simulink model "HM_to_Unity_2013a"  (R2013a)
settings: Solver=FixedStepDiscrete  StartTime=0.0  StopTime=Inf  FixedStep=0.0004  RelTol=1e-3
InitFcn:
  | SampleTime = 0.0004;
  | sampleTime = 0.0004;
undefined symbols (not defined in the file or in its folder): DiscIntNeverNeededParam
libraries: simulink x26, dspsigops x10, xpcmeasurementcomputinglib x7, xpclib x6, dspmtrx3 x4, etargetslib x2, hm_iointerface_lib x2, hm_control_lib x2, sensors_jr3_lib x1
(part 1 of 2)
settings Model: SimulationMode=external  BufferReuse=off  Creator=janezp  LastModifiedBy=student
settings DataIOCC: LimitDataPoints=off  MaxDataPoints=5000000  SaveFormat=Structure  SignalLoggingSaveFormat=ModelDataLogs  SignalLogging=off  SaveTime=off
settings OptimizationCC: BlockReduction=off  OptimizeBlockIOStorage=off  BufferReuse=off  ExpressionFolding=off  ExpressionDepthLimit=2147483647  LocalBlockOutputs=off  InitFltsAndDblsToZero=on
settings DebuggingCC: SaveWithParameterizedLinksMsg=none  SignalResolutionControl=TryResolveAllWithWarning  MultiTaskDSMMsg=warning  MultiTaskCondExecSysMsg=none  FcnCallInpInsideContextMsg=UseLocalSettings  StrictBusMsg=None
settings HardwareCC: ProdIntDivRoundTo=Zero  ProdEndianess=LittleEndian  ProdHWDeviceType=Generic->32-bit x86 compatible
settings RTWCC: SystemTargetFile=xpctarget.tlc  TemplateMakefile=xpc_default_tmf  Description=xPC Target  ProcessScript=xpctarget_make_rtw_hook  IncludeERTFirstTime=on  RTWCompilerOptimization=On
settings xpcTargetCC: TargetFcnLib=ansi_tfl_table_tmw.mat  CodeReplacementLibrary=XPC_BLAS  ParMdlRefBuildCompliant=on  ConcurrentExecutionCompliant=on  CombineSignalStateStructs=off  MATLABClassNameForMDSCustomization=xpcAperiodicCustomization  GRTInterface=on  GenerateAllocFcn=off  RL32LogTETModifier=off  RL32LogBufSizeModifier=5000000  xPCTaskExecutionProfile=off  xPCRL32EventNumber=5000  xPCLoadParamSetFile=off  xPCConcurrentTasks=off  xPCEnableSFAnimation=off

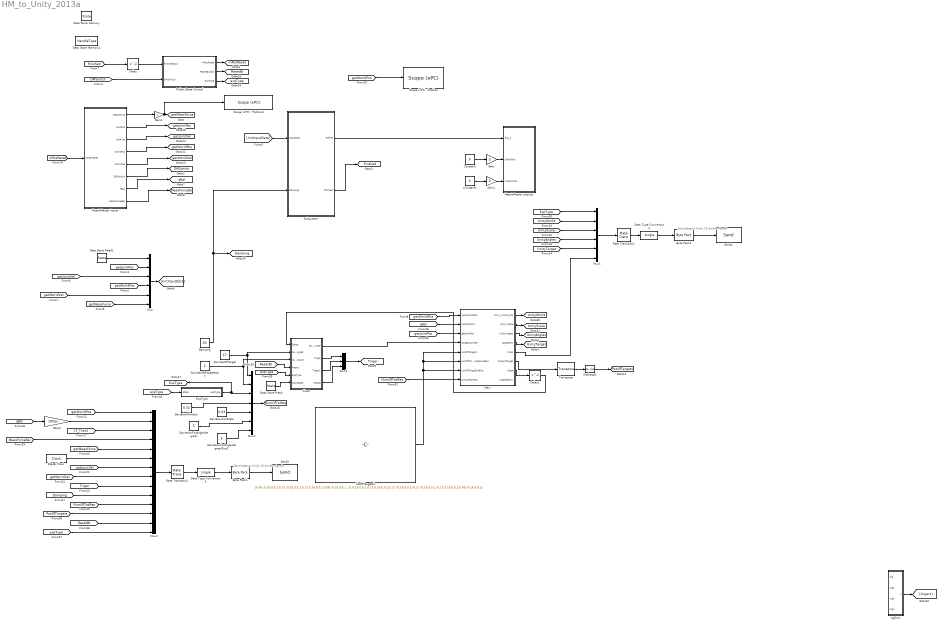
== system HM_to_Unity_2013a ==
  note: Send data to Unity
      | 16 double signals
  note: Send data to Unity
      | 16 double signals
  Byte Pack1 : etargetslib/Byte Pack  datatypes={'single'}  byteAlign=1
  Byte Pack2 : etargetslib/Byte Pack  datatypes={'single'}  byteAlign=1
  Chart : Stateflow chart  TreatAsAtomicUnit=on
  Constant : Constant  Value=0  SampleTime=-1
  Constant1 : Constant  Value=0  SampleTime=-1
  Damping : Constant  Value=40
  Data Store Memory : DataStoreMemory  DataStoreName=State  ReadBeforeWriteMsg=warning  WriteAfterWriteMsg=warning  WriteAfterReadMsg=warning
  Data Store Memory1 : DataStoreMemory  DataStoreName=HandleType  ReadBeforeWriteMsg=warning  WriteAfterWriteMsg=warning  WriteAfterReadMsg=warning
  Data Store Read : DataStoreRead  DataStoreName=State
  Data Store Read1 : DataStoreRead  DataStoreName=State  SampleTime=SampleTime
  Data Type Conversion2 : DataTypeConversion  OutDataTypeStr=single
  Data Type Conversion3 : DataTypeConversion  OutDataTypeStr=single
  Delay : Delay  DelayLength=1  InitialCondition=0
  Delay1 : Delay  DelayLength=1  InitialCondition=0  SampleTime=0.0004
  DeviationForAngle(degree) : Constant  Value=5
  DeviationForAngle(degree)Exp2 : Constant  Value=5
  DeviationForScale : Constant  Value=0.03
  DeviationWindow : Constant  Value=0.02
  Digital Clock : DigitalClock  SampleTime=0.0004
  ExpType : Stateflow chart  TreatAsAtomicUnit=on
  Gain : Gain  Gain=0
  Gain1 : Gain  Gain=0
  Gain2 : Gain
  Gain3 : Gain  Gain=180/pi
  HapticMaster inputs : Subsystem
  HapticMaster outputs : Subsystem
  ListOfTargets1 : Constant  Value=[0.00,-0.16,0,0,1;0.17,-0.16,0,0,1;0.17,0.16,0,0,1;0.00,-0.16,0,0,1;-0.17,-0.16,0,0,1;0.17,-0.16,0,0,1;0.00,-0.16,0,0,1;-0.17,0.16,0,0,1;-0.17,-0.16,0,0,1;0.00,-0.16,0,0,1;0.00,0.16,0,0,1;0.00,-0.16,0,0,1;0.17,0.16,0,0,1;0.17,-0.16,0,0,1;-0.17,-0.16,0,0,1;-0.17,0.16,0,0,1;0.00,-0.16,0,0,1]
  Main : MATLAB Function  TreatAsAtomicUnit=on
  Mux : Mux  Inputs=6
  Mux1 : Mux  Inputs=6
  Mux2 : Mux  Inputs=14
  Mux3 : Mux  Inputs=3
  Mux4 : Mux  Inputs=7
  NumberOfRepeatation : Constant  Value=2
  NumberOfTarget : Constant  Value=17
  Rate Transition1 : RateTransition  OutPortSampleTime=0.02
  Rate Transition2 : RateTransition  OutPortSampleTime=0.01
  Reshape1 : Reshape
  Robot State Control : Subsystem
  Scope (xPC)  Position : xpclib/Misc./Scope (xPC)   scopeno=1  scopetype=Target  autostart=on  viewmode=Numerical  formatstr='Position x: %8.3f m,Position y: %8.3f m,Position z: %8.3f m'  grid=on  ylimits=[0,0]  nosamples=250  noprepostsamples=0  interleave=1  triggermode=FreeRun  triggersignal=1  trigsignalfromport=off  triggerlevel=0.0  triggerslope=Either  triggerscope=1  triggersample=0  filename=data.dat  mode=Lazy  writesize=512  autorestart=off  dynamicfilemode=off  maxwritefilesize=512*1024^2
  Scope (xPC)  Position1 : xpclib/Misc./Scope (xPC)   scopeno=4  scopetype=Target  autostart=on  viewmode=Numerical  formatstr='Fx: %8.3f N,Fy: %8.3f N,Fz: %8.3f N'  grid=on  ylimits=[0,0]  nosamples=250  noprepostsamples=0  interleave=1  triggermode=FreeRun  triggersignal=1  trigsignalfromport=off  triggerlevel=0.0  triggerslope=Either  triggerscope=1  triggersample=0  filename=data.dat  mode=Lazy  writesize=512  autorestart=off  dynamicfilemode=off  maxwritefilesize=512*1024^2
  Send1 : xpclib/UDP/Send  ipAddress=192.168.65.40  ipPort=25008  localPort=-1  vblLen=off  sampletime=0.02
  Send2 : xpclib/UDP/Send  ipAddress=192.168.65.40  ipPort=25010  localPort=-1  vblLen=off  sampletime=0.01
  Subsystem : Subsystem
  Transpose : dspmtrx3/Transpose  Hermitian=off  overflowFlag=off
  "trgSum " : MATLAB Function  TreatAsAtomicUnit=on
  tag scope: DMSwitch=global, Damping=global, ExpType=global, MeasForceBal=global, NumOfTatRep=global, PosOfTargets=global, ResetBt=global, Triger=global, UnityAngles=global, UnityScale=global, UnityTarget=global, UnityWorld=global, expType=global, finished=global, getJointPos=global, getJointVel=global, getMeasForce=global, getWorldPos=global, getWorldVel=global, inPosReset=global, qBal=global
  wires:
  [getWorldPos] -> Mux/4
  [getJointPos] -> Mux/2
  Data Store Read1/1 -> Mux/1
  Mux/1 -> [InitInputData]
  [getWorldPos] -> Scope (xPC)  Position/1
  HapticMaster inputs/1(MeasForce) -> Gain2/1
  HapticMaster inputs/3(JointVel) -> [getJointVel]
  HapticMaster inputs/5(WorldVel) -> [getWorldVel]
  Delay/1 -> Robot State Control/1(finishedTask)
  [DMSwitch] -> Robot State Control/2(DMSwitch)
  Robot State Control/1(inPosReset) -> [inPosReset]
  HapticMaster inputs/6(DMSwitch) -> [DMSwitch]
  [inPosReset] -> HapticMaster inputs/1(inPosReset)
  [getMeasForce] -> Mux/6
  [InitInputData] -> Subsystem/1(InputData)
  Subsystem/2(finished) -> [finished]
  [finished] -> Delay/1
  Subsystem/1(RefVel) -> HapticMaster outputs/1(dot_q)
  HapticMaster inputs/8(MeasForceBal) -> [MeasForceBal]
  HapticMaster inputs/7(qBal) -> [qBal]
  Gain2/1 -> Scope (xPC)  Position1/1, [getMeasForce]
  HapticMaster inputs/4(WorldPos) -> [getWorldPos]
  HapticMaster inputs/2(JointPos) -> [getJointPos]
  [getJointVel] -> Mux/3
  [getWorldVel] -> Mux/5
  "trgSum "/1(y) -> [trigers]
  Rate Transition1/1 -> Data Type Conversion2/1
  Data Type Conversion2/1 -> Byte Pack2/1
  Mux1/1 -> Rate Transition1/1
  Byte Pack2/1 -> Send1/1
  [getWorldPos] -> Main/1(inputWorldPos)
  Main/1(Unity_World_Pos) -> [UnityWorld]
  [UnityWorld] -> Mux1/2
  Main/2(Unity_Scale) -> [UnityScale]
  [UnityScale] -> Mux1/3
  Main/3(UnityAngles) -> [UnityAngles]
  [UnityAngles] -> Mux1/4
  Chart/1(TargetNumber) -> Main/4(TargetNumber)
  Main/4(TargetPos) -> [UnityTarget]
  [UnityTarget] -> Mux1/5
  Main/7(State) -> Delay1/1
  Delay1/1 -> Chart/1(State)
  Main/5(Color) -> Mux1/6
  NumberOfRepeatation/1 -> Mux4/2, Chart/3(NumberOfRepetation)
  NumberOfTarget/1 -> Chart/2(NumOfTarget), Mux4/1
  [getWorldPos] -> Mux2/1
  [qBal] -> Gain3/1
  Gain3/1 -> Mux2/2
  [F_Traw] -> Mux2/3
  [MeasForceBal] -> Mux2/4
  [getMeasForce] -> Mux2/5
  Digital Clock/1 -> Mux2/6
  [getJointVel] -> Mux2/7
  [getWorldVel] -> Mux2/8
  Rate Transition2/1 -> Data Type Conversion3/1
  Byte Pack1/1 -> Send2/1
  Data Type Conversion3/1 -> Byte Pack1/1
  Mux2/1 -> Rate Transition2/1
  [qBal] -> Main/2(inputMotors)
  Chart/2(Triger) -> Mux3/1
  Chart/3(Triger2) -> Mux3/2
  Mux3/1 -> [Triger]
  [Triger] -> Mux2/9
  Mux4/1 -> [NumOfTatRep]
  [NumOfTatRep] -> Main/8(NumOfTarRep)
  [Damping] -> Mux2/10
  Damping/1 -> [Damping], Subsystem/2("Damping ")
  Chart/4(repeat) -> Mux3/3
  [NumOfTatRep] -> Mux2/11
  [PosOfTargets] -> Mux2/12
  Reshape1/1 -> [PosOfTargets]
  Transpose/1 -> Reshape1/1
  Main/6(OutputTarget) -> Transpose/1
  DeviationWindow/1 -> Mux4/4
  [ExpType] -> Mux1/1
  DeviationForScale/1 -> Mux4/5
  DeviationForAngle(degree)/1 -> Mux4/6
  DeviationForAngle(degree)Exp2/1 -> Mux4/7
  [getJointPos] -> Main/3(getJointPos)
  Robot State Control/2("ResetButton ") -> [ResetBt]
  [ResetBt] -> Chart/4(Reset)
  Robot State Control/3(expType) -> [expType]
  [expType] -> ExpType/1(State)
  [expType] -> Chart/5(ExpType)
  [ResetBt] -> Mux2/13
  [expType] -> Mux2/14
  ExpType/1(expType) -> Mux4/3, [ExpType]
  Data Store Read/1 -> Chart/6(MainState)
  ListOfTargets1/1 -> Main/7(ListOfTarget3rdExp), Main/5(ListOfTargets), Main/6(ListOfTargetsForSecondExp)
  Gain/1 -> HapticMaster outputs/2(UMaliMot)
  Constant/1 -> Gain/1
  Constant1/1 -> Gain1/1
  Gain1/1 -> HapticMaster outputs/3(UVelikiMot)

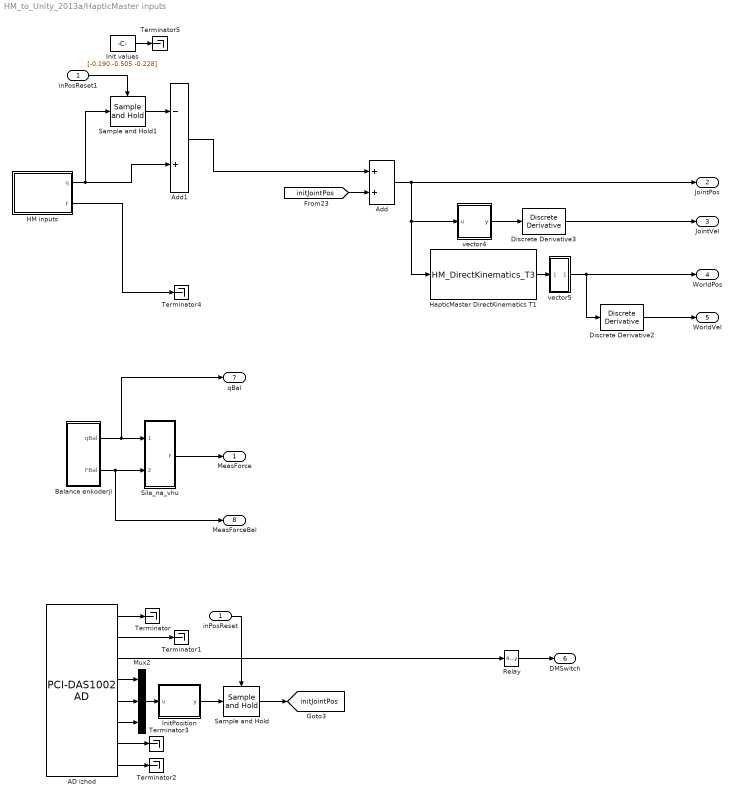
== system HM_to_Unity_2013a/HapticMaster inputs ==
  inPosReset : Inport
  AD izhod : xpcmeasurementcomputinglib/A//D/PCI-DAS1002 AD  channel=8  range=+-10V  mux=Differential (8 channels)  sampletime=-1  slot=-1
  Add : Sum
  Add1 : Sum  Inputs=-+
  Balanca enkoderji : Subsystem
  Discrete Derivative2 : simulink/Discrete/Discrete Derivative  gainval=1.0  ICPrevScaledInput=0.0  InputProcessing=Inherited  OutMin=[]  OutMax=[]  OutDataType=sfix(16)  OutScaling=2^-10  DoSatur=off
  Discrete Derivative3 : simulink/Discrete/Discrete Derivative  gainval=1.0  ICPrevScaledInput=0.0  InputProcessing=Inherited  OutMin=[]  OutMax=[]  OutDataType=sfix(16)  OutScaling=2^-10  DoSatur=off
  HM inputs : Subsystem  mask(HapticMaster input driver){gimbal_out=off, force_out=on}
      mask prompts: gimbal_out "Show gimbal output port"; force_out "Show force output port"
      mask help:
      | q - robot joint positions
      | q_gimbal - gimbal joint positions
      | F - end-effector forces
      mask init:
      | set_param(gcb', 'LinkStatus', 'none')
      | 
      | port = 2;
      | current_block = gcb;
      | 
      | if (gimbal_out == 1)
      |     block = find_system(current_block, 'FollowLinks', 'on', 'LookUnderMasks', 'on', 'Name', 'q_gimbal', 'BlockType', 'Outport');
      |     if isempty(block)    
      |         replace_block(current_block,'Name','q_gimbal','Outport','noprompt');
      |         set_param([current_block,'/q_gimbal'], 'Port', int2str(port));
      |     end
      |     port = port + 1;
      | end
      | 
      | if (gimbal_out == 0)
      |     replace_block(current_block,'Name','q_gimbal','Terminator','noprompt');
      | end
      | 
      | if (force_out == 1)
      |     block = find_system(current_block, 'FollowLinks', 'on', 'LookUnderMasks', 'on', 'Name', 'F', 'BlockType', 'Outport');
      |     if isempty(block)    
      |         replace_block(current_block,'Name','F','Outport','noprompt');
      |         set_param([current_block,'/F'], 'Port', int2str(port));
      |     end
      |     port = port + 1;
      | end
      | 
      | if (force_out == 0)
      |     replace_block(current_block,'Name','F','Terminator','noprompt');
      | end
  HapticMaster DirectKinematics T1 : S-Function  InitFcn=try, set_param(gcb,'FunctionName','HM_DirectKinematics_T3'), end  FunctionName=HM_DirectKinematics_T3  SFunctionModules=HM_DirectKinematics_T3_wrapper  EnableBusSupport=off  mask(S-Function Builder){}
      mask help: The S-Function Builder block creates a wrapper C-MEX S-function from your supplied C code with multiple input ports, output ports, and a variable number of scalar, vector, or matrix parameters. The input and output ports can propagate Simulink built-in data types, fixed-point datatypes, complex, frame, 1-D, and 2-D signals. This block also supports discrete and continuous states of type real. You can optionally have the block generate a TLC file to be used with Real-Time Workshop for code generation.
      mask init:
      | val = [[.9  0.75 0.75 1 1 .9 .9 1]',[1 1 0.75 0.75 .9 .9 1 .9]'];try , sys = get_param(gcb,'SfunBuilderFcnName');if isempty(sys), sys = get_param(gcb,'FunctionName'); end,catch, sys = get_param(gcb,'FunctionName'); end
      settings: CopyFcn=set_param(gcbh,'LinkStatus','none')  PreSaveFcn=try, set_param(gcb,'FunctionName','HM_DirectKinematics_T3'), end  OpenFcn=sfunctionwizard(gcbh)
      mask Display: plot(val(:,1),val(:,2)),disp(sys), port_label('input',1,'q'), port_label('output',1,'x')
  Init values : Constant  Value=[-0.190 -0.505 -0.228]
  InitPosition : MATLAB Function  TreatAsAtomicUnit=on
  Mux2 : Mux  Inputs=3
  Relay : Relay  OnSwitchValue=4.0  OffSwitchValue=2.5
  Sample and Hold : dspsigops/Sample and Hold  trig=Rising edge  initCond=[-0.190 -0.504 -0.228]  latchinput=off
  Sample and Hold1 : dspsigops/Sample and Hold  trig=Rising edge  initCond=[-0.190 -0.504 -0.228]  latchinput=off
  Sila_na_vhu : Subsystem
  Terminator{,1..5} (6 alike) : Terminator
  inPosReset1 : InportShadow
  vector4 : MATLAB Function  TreatAsAtomicUnit=on
  vector5 : MATLAB Function  TreatAsAtomicUnit=on
  MeasForce : Outport
  JointPos : Outport  Port=2
  JointVel : Outport  Port=3
  WorldPos : Outport  Port=4
  WorldVel : Outport  Port=5
  DMSwitch : Outport  Port=6
  qBal : Outport  Port=7
  MeasForceBal : Outport  Port=8
  tag scope: initJointPos=global
  wires:
  Discrete Derivative2/1 -> WorldVel/1
  Add/1 -> HapticMaster DirectKinematics T1/1, vector4/1(u), JointPos/1
  Discrete Derivative3/1 -> JointVel/1
  vector4/1(y) -> Discrete Derivative3/1
  vector5/1(y) -> WorldPos/1, Discrete Derivative2/1
  HapticMaster DirectKinematics T1/1 -> vector5/1(u)
  AD izhod/3 -> Relay/1
  Relay/1 -> DMSwitch/1
  AD izhod/4 -> Mux2/1
  AD izhod/5 -> Mux2/2
  AD izhod/6 -> Mux2/3
  Mux2/1 -> InitPosition/1(u)
  InitPosition/1(y) -> Sample and Hold/1
  Sample and Hold/1 -> [initJointPos]
  inPosReset/1 -> Sample and Hold/Trigger
  AD izhod/1 -> Terminator/1
  AD izhod/2 -> Terminator1/1
  AD izhod/8 -> Terminator2/1
  AD izhod/7 -> Terminator3/1
  HM inputs/2(F) -> Terminator4/1
  Add1/1 -> Add/1
  [initJointPos] -> Add/2
  Init values/1 -> Terminator5/1
  HM inputs/1(q) -> Sample and Hold1/1, Add1/2
  Sample and Hold1/1 -> Add1/1
  inPosReset1/1 -> Sample and Hold1/Trigger
  Balanca enkoderji/2(FBal) -> MeasForceBal/1, Sila_na_vhu/2(Fbal)
  Balanca enkoderji/1(qBal) -> qBal/1, Sila_na_vhu/1(qBal)
  Sila_na_vhu/1(F) -> MeasForce/1

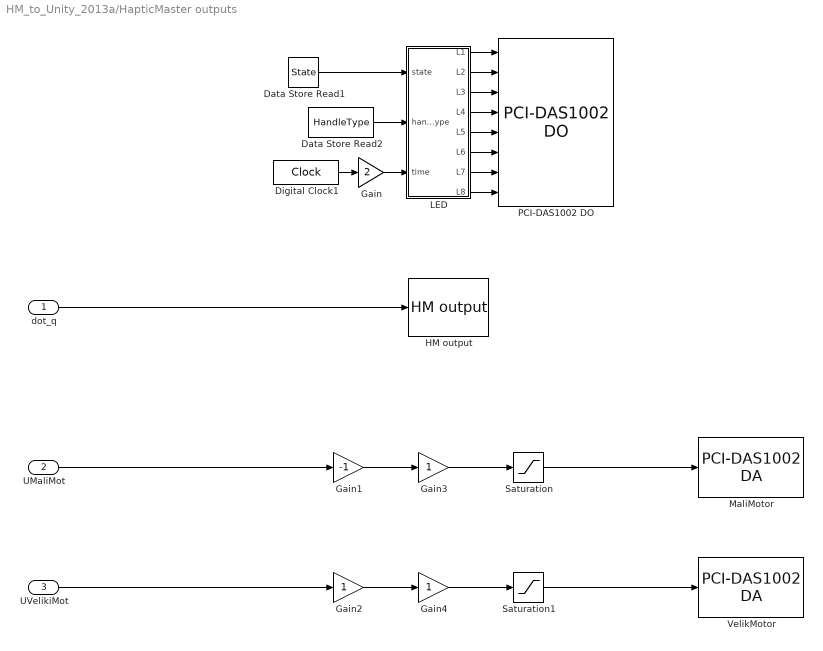
== system HM_to_Unity_2013a/HapticMaster outputs ==
  dot_q : Inport
  UMaliMot : Inport  Port=2
  UVelikiMot : Inport  Port=3
  Data Store Read1 : DataStoreRead  DataStoreName=State  SampleTime=SampleTime
  Data Store Read2 : DataStoreRead  DataStoreName=HandleType  SampleTime=SampleTime
  Digital Clock1 : DigitalClock  SampleTime=-1
  Gain : Gain  Gain=2
  Gain1 : Gain  Gain=-1
  Gain2 : Gain
  Gain3 : Gain
  Gain4 : Gain
  HM output : hm_iointerface_lib/HM output
  LED : MATLAB Function  TreatAsAtomicUnit=on
  MaliMotor : xpcmeasurementcomputinglib/D//A/PCI-DAS1002 DA  channel=[1]  range=[-10]  reset=[1]  initValue=[0]  sampletime=0.0004  pci_dev=-1
  PCI-DAS1002 DO : xpcmeasurementcomputinglib/Digital Output/PCI-DAS1002 DO  channel=[1 2 3 4 5 6 7 8]  port=C  reset=[1 1 1 1 1 1 1 1]  initValue=[0 0 0 0 0 0 0 0]  chip=1  sampletime=-1  slot=-1
  Saturation : Saturate  UpperLimit=10  LowerLimit=-10
  Saturation1 : Saturate  UpperLimit=10  LowerLimit=-10
  VelikMotor : xpcmeasurementcomputinglib/D//A/PCI-DAS1002 DA  channel=[2]  range=[-10]  reset=[1]  initValue=[0]  sampletime=0.0004  pci_dev=-1
  wires:
  dot_q/1 -> HM output/1
  Gain/1 -> LED/3(time)
  LED/4(L4) -> PCI-DAS1002 DO/4
  LED/2(L2) -> PCI-DAS1002 DO/2
  LED/5(L5) -> PCI-DAS1002 DO/5
  LED/8(L8) -> PCI-DAS1002 DO/8
  Data Store Read1/1 -> LED/1(state)
  LED/7(L7) -> PCI-DAS1002 DO/7
  LED/6(L6) -> PCI-DAS1002 DO/6
  LED/3(L3) -> PCI-DAS1002 DO/3
  LED/1(L1) -> PCI-DAS1002 DO/1
  Digital Clock1/1 -> Gain/1
  UMaliMot/1 -> Gain1/1
  UVelikiMot/1 -> Gain2/1
  Saturation/1 -> MaliMotor/1
  Saturation1/1 -> VelikMotor/1
  Gain1/1 -> Gain3/1
  Gain2/1 -> Gain4/1
  Data Store Read2/1 -> LED/2(handleType)
  Gain3/1 -> Saturation/1
  Gain4/1 -> Saturation1/1

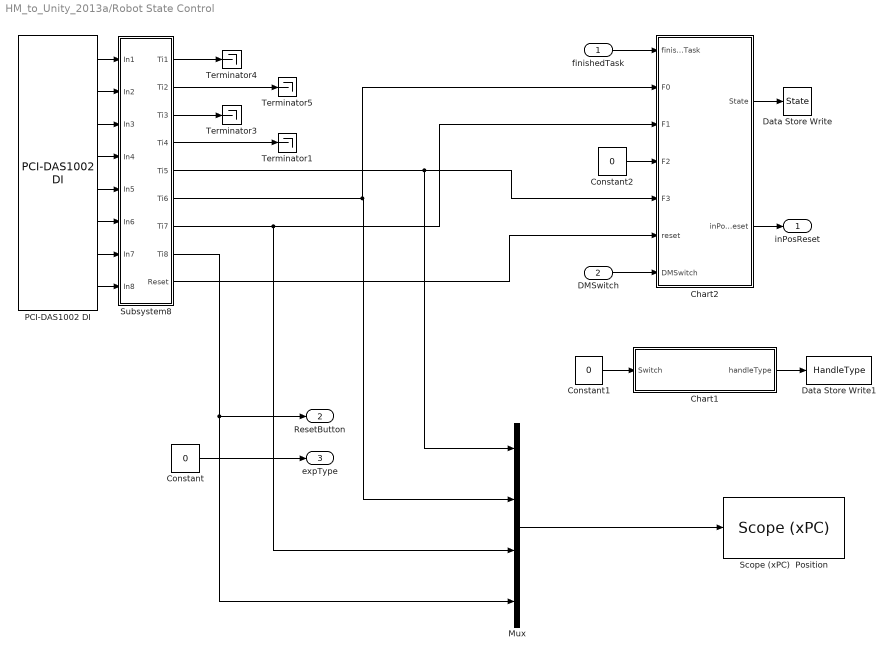
== system HM_to_Unity_2013a/Robot State Control ==
  finishedTask : Inport
  DMSwitch : Inport  Port=2
  Chart1 : Stateflow chart  TreatAsAtomicUnit=on
  Chart2 : Stateflow chart  TreatAsAtomicUnit=on
  Constant : Constant  Value=0
  Constant1 : Constant  Value=0
  Constant2 : Constant  Value=0
  Data Store Write : DataStoreWrite  DataStoreName=State  SampleTime=SampleTime
  Data Store Write1 : DataStoreWrite  DataStoreName=HandleType  SampleTime=SampleTime
  Mux : Mux
  PCI-DAS1002 DI : xpcmeasurementcomputinglib/Digital Input/PCI-DAS1002 DI  channel=[1 2 3 4 5 6 7 8]  port=A  chip=1  sampletime=-1  slot=-1
  Scope (xPC)  Position : xpclib/Misc./Scope (xPC)   scopeno=2  scopetype=Target  autostart=on  viewmode=Numerical  formatstr='T5: %8.1f, T6: %8.1f, T7: %8.1f, T8: %8.1f'  grid=on  ylimits=[0,0]  nosamples=250  noprepostsamples=0  interleave=1  triggermode=FreeRun  triggersignal=1  trigsignalfromport=off  triggerlevel=0.0  triggerslope=Either  triggerscope=1  triggersample=0  filename=data.dat  mode=Lazy  writesize=512  autorestart=off  dynamicfilemode=off  maxwritefilesize=512*1024^2
  Subsystem8 : Subsystem
  Terminator{1,3..5} (4 alike) : Terminator
  inPosReset : Outport
  "ResetButton " : Outport  Port=2
  expType : Outport  Port=3
  wires:
  Subsystem8/7(Ti7) -> Chart2/3(F1), Mux/3
  finishedTask/1 -> Chart2/1(finishedTask)
  Chart2/1(State) -> Data Store Write/1
  Subsystem8/5(Ti5) -> Mux/1, Chart2/5(F3)
  PCI-DAS1002 DI/4 -> Subsystem8/4(In4)
  PCI-DAS1002 DI/8 -> Subsystem8/8(In8)
  PCI-DAS1002 DI/7 -> Subsystem8/7(In7)
  PCI-DAS1002 DI/2 -> Subsystem8/2(In2)
  Chart2/2(inPosReset) -> inPosReset/1
  PCI-DAS1002 DI/3 -> Subsystem8/3(In3)
  Subsystem8/9(Reset) -> Chart2/6(reset)
  Subsystem8/6(Ti6) -> Chart2/2(F0), Mux/2
  PCI-DAS1002 DI/6 -> Subsystem8/6(In6)
  DMSwitch/1 -> Chart2/7(DMSwitch)
  PCI-DAS1002 DI/5 -> Subsystem8/5(In5)
  PCI-DAS1002 DI/1 -> Subsystem8/1(In1)
  Subsystem8/1(Ti1) -> Terminator4/1
  Chart1/1(handleType) -> Data Store Write1/1
  Constant/1 -> expType/1
  Subsystem8/3(Ti3) -> Terminator3/1
  Constant1/1 -> Chart1/1(Switch)
  Subsystem8/4(Ti4) -> Terminator1/1
  Subsystem8/8(Ti8) -> "ResetButton "/1, Mux/4
  Mux/1 -> Scope (xPC)  Position/1
  Subsystem8/2(Ti2) -> Terminator5/1
  Constant2/1 -> Chart2/4(F2)

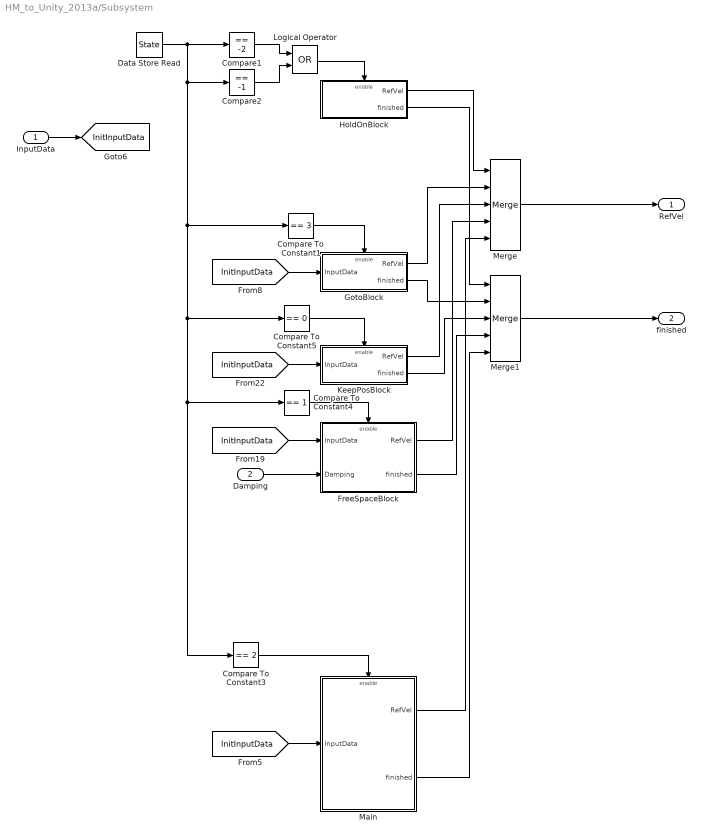
== system HM_to_Unity_2013a/Subsystem ==
  InputData : Inport
  "Damping " : Inport  Port=2
  Compare To Constant1 : simulink/Logic and Bit Operations/Compare To Constant  relop===  const=3  OutDataTypeStr=boolean  ZeroCross=off
  Compare To Constant3 : simulink/Logic and Bit Operations/Compare To Constant  relop===  const=2  OutDataTypeStr=boolean  ZeroCross=off
  Compare To Constant4 : simulink/Logic and Bit Operations/Compare To Constant  relop===  const=1  OutDataTypeStr=boolean  ZeroCross=off
  Compare To Constant5 : simulink/Logic and Bit Operations/Compare To Constant  relop===  const=0  OutDataTypeStr=boolean  ZeroCross=off
  Compare1 : simulink/Logic and Bit Operations/Compare To Constant  relop===  const=-2  OutDataTypeStr=boolean  ZeroCross=off
  Compare2 : simulink/Logic and Bit Operations/Compare To Constant  relop===  const=-1  OutDataTypeStr=boolean  ZeroCross=off
  Data Store Read : DataStoreRead  DataStoreName=State  SampleTime=SampleTime
  FreeSpaceBlock : Subsystem  TreatAsAtomicUnit=on
  GotoBlock : Subsystem  TreatAsAtomicUnit=on
  HoldOnBlock : Subsystem  TreatAsAtomicUnit=on
  KeepPosBlock : Subsystem  TreatAsAtomicUnit=on
  Logical Operator : Logic  Operator=OR  AllPortsSameDT=off  OutDataTypeStr=boolean
  Main : Subsystem  TreatAsAtomicUnit=on
  Merge : Merge  Inputs=5  InitialOutput=[0 0 0]
  Merge1 : Merge  Inputs=5  InitialOutput=0
  RefVel : Outport
  finished : Outport  Port=2
  tag scope: InitInputData=global
  wires:
  [InitInputData] -> GotoBlock/1(InputData)
  HoldOnBlock/1(RefVel) -> Merge/1
  Main/1(RefVel) -> Merge/5
  Main/2(finished) -> Merge1/5
  [InitInputData] -> FreeSpaceBlock/1(InputData)
  GotoBlock/1(RefVel) -> Merge/2
  Compare To Constant3/1 -> Main/Enable
  Compare To Constant4/1 -> FreeSpaceBlock/Enable
  [InitInputData] -> Main/1(InputData)
  Compare To Constant1/1 -> GotoBlock/Enable
  HoldOnBlock/2(finished) -> Merge1/1
  FreeSpaceBlock/1(RefVel) -> Merge/4
  FreeSpaceBlock/2(finished) -> Merge1/4
  Compare2/1 -> Logical Operator/2
  KeepPosBlock/1(RefVel) -> Merge/3
  Data Store Read/1 -> Compare To Constant1/1, Compare To Constant5/1, Compare To Constant3/1, Compare To Constant4/1, Compare2/1, Compare1/1
  GotoBlock/2(finished) -> Merge1/2
  Compare To Constant5/1 -> KeepPosBlock/Enable
  Compare1/1 -> Logical Operator/1
  [InitInputData] -> KeepPosBlock/1(InputData)
  KeepPosBlock/2(finished) -> Merge1/3
  Logical Operator/1 -> HoldOnBlock/Enable
  Merge/1 -> RefVel/1
  Merge1/1 -> finished/1
  InputData/1 -> [InitInputData]
  "Damping "/1 -> FreeSpaceBlock/2("Damping ")

== system HM_to_Unity_2013a/HapticMaster inputs/Balanca enkoderji ==
  Desna roka : Subsystem
  Gain : Gain  Gain=180/pi
  Gain3 : Gain  Gain=(-2*pi)/(4*500*26*2)
  Gain4 : Gain  Gain=(-2*pi)/(4*1024*26)
  Mali motor : xpcmeasurementcomputinglib/Incremental Encoder/PCI-QUAD04   channel=2  resetmode=off  polarity=Positive Index  mode=Normal  limit=5000  range=-2^23...+2^23-1  speed=4x  prescale=0  ts=0.0004  convbaseaddr=-1
  Mux : Mux  Inputs=2
  Scope (xPC)  Position2 : xpclib/Misc./Scope (xPC)   scopeno=3  scopetype=Target  autostart=on  viewmode=Numerical  formatstr='Q1: %8.3f,Q2: %8.3f'  grid=on  ylimits=[0,0]  nosamples=250  noprepostsamples=0  interleave=1  triggermode=FreeRun  triggersignal=1  trigsignalfromport=off  triggerlevel=0.0  triggerslope=Either  triggerscope=1  triggersample=0  filename=data.dat  mode=Lazy  writesize=512  autorestart=off  dynamicfilemode=off  maxwritefilesize=512*1024^2
  Sile na rockah : MATLAB Function  TreatAsAtomicUnit=on
  Step : Step  Time=0.0004  SampleTime=0.0004
  Velik motor : xpcmeasurementcomputinglib/Incremental Encoder/PCI-QUAD04   channel=1  resetmode=off  polarity=Positive Index  mode=Normal  limit=5000  range=-2^23...+2^23-1  speed=4x  prescale=0  ts=0.0004  convbaseaddr=-1
  qBal : Outport
  FBal : Outport  Port=2
  wires:
  Desna roka/1(FT) -> Sile na rockah/1(Fd)
  Step/1 -> Desna roka/1(Rst)
  Mux/1 -> Gain/1, qBal/1
  Gain4/1 -> Mux/2
  Gain3/1 -> Mux/1
  Velik motor/1 -> Gain4/1
  Mali motor/1 -> Gain3/1
  Sile na rockah/1(Fdo) -> FBal/1
  Gain/1 -> Scope (xPC)  Position2/1

== system HM_to_Unity_2013a/HapticMaster inputs/HM inputs ==
  Driver outputs : hm_iointerface_lib/Absolete/Driver outputs  Channels=0
  q_gimbal : Terminator
  q : Outport
  F : Outport  Port=2
  wires:
  Driver outputs/3 -> q_gimbal/1
  Driver outputs/2 -> q/1
  Driver outputs/1 -> F/1

== system HM_to_Unity_2013a/HapticMaster inputs/Sila_na_vhu ==
  qBal : Inport
  Fbal : Inport  Port=2
  Demux1 : Demux  Outputs=2
  Sila na vrhu : MATLAB Function  TreatAsAtomicUnit=on
  F : Outport
  wires:
  Fbal/1 -> Sila na vrhu/3(Fd)
  Demux1/2 -> Sila na vrhu/2(rot_velik)
  Demux1/1 -> Sila na vrhu/1(rot_mali)
  qBal/1 -> Demux1/1
  Sila na vrhu/1(F) -> F/1

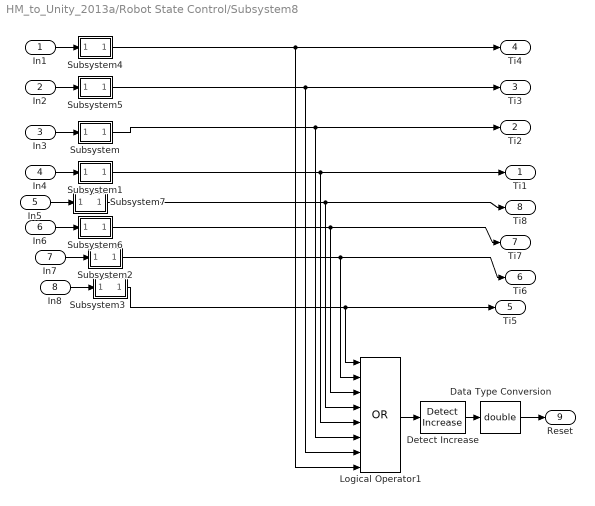
== system HM_to_Unity_2013a/Robot State Control/Subsystem8 ==
  In1 : Inport
  In2 : Inport  Port=2
  In3 : Inport  Port=3
  In4 : Inport  Port=4
  In5 : Inport  Port=5
  In6 : Inport  Port=6
  In7 : Inport  Port=7
  In8 : Inport  Port=8
  Data Type Conversion : DataTypeConversion  OutDataTypeStr=double
  Detect Increase : simulink/Logic and Bit Operations/Detect Increase  vinit=0.0  InputProcessing=Inherited  OutDataTypeStr=uint8
  Logical Operator1 : Logic  Operator=OR  Inputs=8  AllPortsSameDT=off  OutDataTypeStr=boolean
  Subsystem : Subsystem
  Subsystem1 : Subsystem
  Subsystem2 : Subsystem
  Subsystem3 : Subsystem
  Subsystem4 : Subsystem
  Subsystem5 : Subsystem
  Subsystem6 : Subsystem
  Subsystem7 : Subsystem
  Ti1 : Outport
  Ti2 : Outport  Port=2
  Ti3 : Outport  Port=3
  Ti4 : Outport  Port=4
  Ti5 : Outport  Port=5
  Ti6 : Outport  Port=6
  Ti7 : Outport  Port=7
  Ti8 : Outport  Port=8
  Reset : Outport  Port=9
  wires:
  Logical Operator1/1 -> Detect Increase/1
  Detect Increase/1 -> Data Type Conversion/1
  Subsystem/1(Out1) -> Ti2/1, Logical Operator1/6
  Subsystem1/1(Out1) -> Ti1/1, Logical Operator1/5
  Subsystem2/1(Out1) -> Ti6/1, Logical Operator1/2
  Subsystem3/1(Out1) -> Ti5/1, Logical Operator1/1
  In1/1 -> Subsystem4/1(In1)
  Subsystem4/1(Out1) -> Ti4/1, Logical Operator1/8
  In2/1 -> Subsystem5/1(In1)
  Subsystem5/1(Out1) -> Ti3/1, Logical Operator1/7
  In3/1 -> Subsystem/1(In1)
  In4/1 -> Subsystem1/1(In1)
  Data Type Conversion/1 -> Reset/1
  In5/1 -> Subsystem7/1(In1)
  Subsystem7/1(Out1) -> Ti8/1, Logical Operator1/4
  In6/1 -> Subsystem6/1(In1)
  Subsystem6/1(Out1) -> Ti7/1, Logical Operator1/3
  In7/1 -> Subsystem2/1(In1)
  In8/1 -> Subsystem3/1(In1)

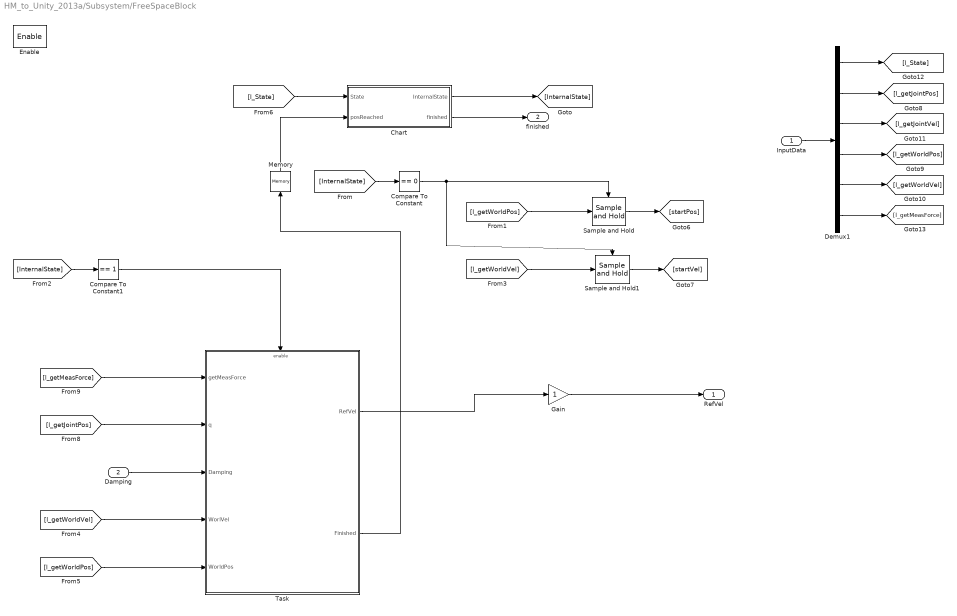
== system HM_to_Unity_2013a/Subsystem/FreeSpaceBlock ==
  InputData : Inport
  "Damping " : Inport  Port=2  PortDimensions=1
  Enable : EnablePort  StatesWhenEnabling=reset
  Chart : Stateflow chart  TreatAsAtomicUnit=on
  Compare To Constant : simulink/Logic and Bit Operations/Compare To Constant  relop===  const=0  OutDataTypeStr=uint8  ZeroCross=off
  Compare To Constant1 : simulink/Logic and Bit Operations/Compare To Constant  relop===  const=1  OutDataTypeStr=uint8  ZeroCross=off
  Demux1 : Demux  Outputs=[1 3 3 3 3 3]
  Gain : Gain
  Memory : Memory  InheritSampleTime=on
  Sample and Hold : dspsigops/Sample and Hold  trig=Rising edge  initCond=[0 0 0]  latchinput=off
  Sample and Hold1 : dspsigops/Sample and Hold  trig=Rising edge  initCond=[0 0 0]  latchinput=off
  Task : Subsystem
  RefVel : Outport  OutputWhenDisabled=reset  InitialOutput=[0 0 0]
  finished : Outport  Port=2  OutDataTypeStr=boolean  OutputWhenDisabled=reset  InitialOutput=0
  wires:
  Sample and Hold/1 -> [startPos]
  [InternalState] -> Compare To Constant/1
  Compare To Constant/1 -> Sample and Hold/Trigger, Sample and Hold1/Trigger
  [InternalState] -> Compare To Constant1/1
  [l_getWorldVel] -> Sample and Hold1/1
  Sample and Hold1/1 -> [startVel]
  Chart/1(InternalState) -> [InternalState]
  [l_getWorldPos] -> Sample and Hold/1
  [l_State] -> Chart/1(State)
  Chart/2(finished) -> finished/1
  Task/2(Finished) -> Memory/1
  Compare To Constant1/1 -> Task/Enable
  Memory/1 -> Chart/2(posReached)
  Gain/1 -> RefVel/1
  Task/1(RefVel) -> Gain/1
  InputData/1 -> Demux1/1
  Demux1/1 -> [l_State]
  Demux1/2 -> [l_getJointPos]
  Demux1/3 -> [l_getJointVel]
  Demux1/4 -> [l_getWorldPos]
  Demux1/5 -> [l_getWorldVel]
  Demux1/6 -> [l_getMeasForce]
  [l_getJointPos] -> Task/2(q)
  [l_getMeasForce] -> Task/1(getMeasForce)
  "Damping "/1 -> Task/3(Damping)
  [l_getWorldVel] -> Task/4("WorlVel ")
  [l_getWorldPos] -> Task/5(WorldPos)

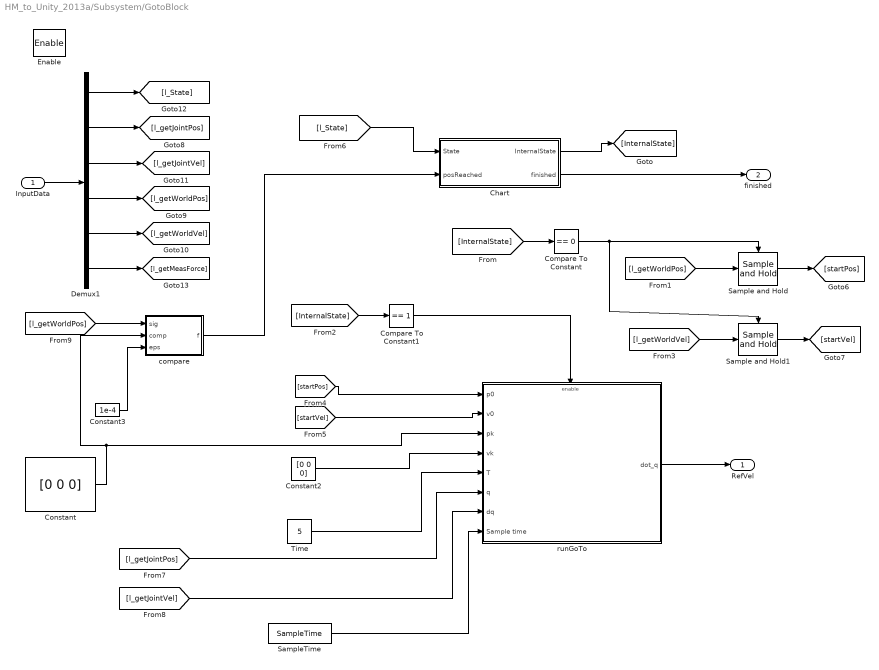
== system HM_to_Unity_2013a/Subsystem/GotoBlock ==
  InputData : Inport
  Enable : EnablePort  StatesWhenEnabling=reset
  Chart : Stateflow chart  TreatAsAtomicUnit=on
  Compare To Constant : simulink/Logic and Bit Operations/Compare To Constant  relop===  const=0  OutDataTypeStr=uint8  ZeroCross=off
  Compare To Constant1 : simulink/Logic and Bit Operations/Compare To Constant  relop===  const=1  OutDataTypeStr=uint8  ZeroCross=off
  Constant : Constant  Value=[0 0 0]
  Constant2 : Constant  Value=[0 0 0]
  Constant3 : Constant  Value=1e-4
  Demux1 : Demux  Outputs=[1 3 3 3 3 3]
  Sample and Hold : dspsigops/Sample and Hold  trig=Rising edge  initCond=[0 0 0]  latchinput=off
  Sample and Hold1 : dspsigops/Sample and Hold  trig=Rising edge  initCond=[0 0 0]  latchinput=off
  SampleTime : Constant  Value=SampleTime  SampleTime=SampleTime
  Time : Constant  Value=5
  compare : MATLAB Function  TreatAsAtomicUnit=on
  runGoTo : Subsystem  TreatAsAtomicUnit=on
  RefVel : Outport  OutputWhenDisabled=reset  InitialOutput=[0 0 0]
  finished : Outport  Port=2  OutDataTypeStr=boolean  OutputWhenDisabled=reset  InitialOutput=0
  wires:
  Sample and Hold/1 -> [startPos]
  [InternalState] -> Compare To Constant/1
  Compare To Constant/1 -> Sample and Hold/Trigger, Sample and Hold1/Trigger
  [InternalState] -> Compare To Constant1/1
  Compare To Constant1/1 -> runGoTo/Enable
  [l_getWorldVel] -> Sample and Hold1/1
  Sample and Hold1/1 -> [startVel]
  [startPos] -> runGoTo/1(p0)
  [startVel] -> runGoTo/2(v0)
  Time/1 -> runGoTo/5(T)
  Constant/1 -> compare/2(comp), runGoTo/3(pk)
  Constant2/1 -> runGoTo/4(vk)
  Chart/1(InternalState) -> [InternalState]
  [l_getWorldPos] -> Sample and Hold/1
  [l_State] -> Chart/1(State)
  runGoTo/1(dot_q) -> RefVel/1
  [l_getJointPos] -> runGoTo/6(q)
  [l_getJointVel] -> runGoTo/7(dq)
  [l_getWorldPos] -> compare/1(sig)
  Constant3/1 -> compare/3(eps)
  Chart/2(finished) -> finished/1
  compare/1(f) -> Chart/2(posReached)
  SampleTime/1 -> runGoTo/8(Sample time)
  InputData/1 -> Demux1/1
  Demux1/1 -> [l_State]
  Demux1/2 -> [l_getJointPos]
  Demux1/3 -> [l_getJointVel]
  Demux1/4 -> [l_getWorldPos]
  Demux1/5 -> [l_getWorldVel]
  Demux1/6 -> [l_getMeasForce]

== system HM_to_Unity_2013a/Subsystem/HoldOnBlock ==
  Enable : EnablePort  StatesWhenEnabling=reset
  Constant1 : Constant  Value=0  OutDataTypeStr=boolean  SampleTime=Inf
  Constant2 : Constant  Value=[0 0 0]  SampleTime=Inf
  RefVel : Outport  OutputWhenDisabled=reset  InitialOutput=[0 0 0]
  finished : Outport  Port=2  OutDataTypeStr=boolean  OutputWhenDisabled=reset  InitialOutput=0
  wires:
  Constant2/1 -> RefVel/1
  Constant1/1 -> finished/1

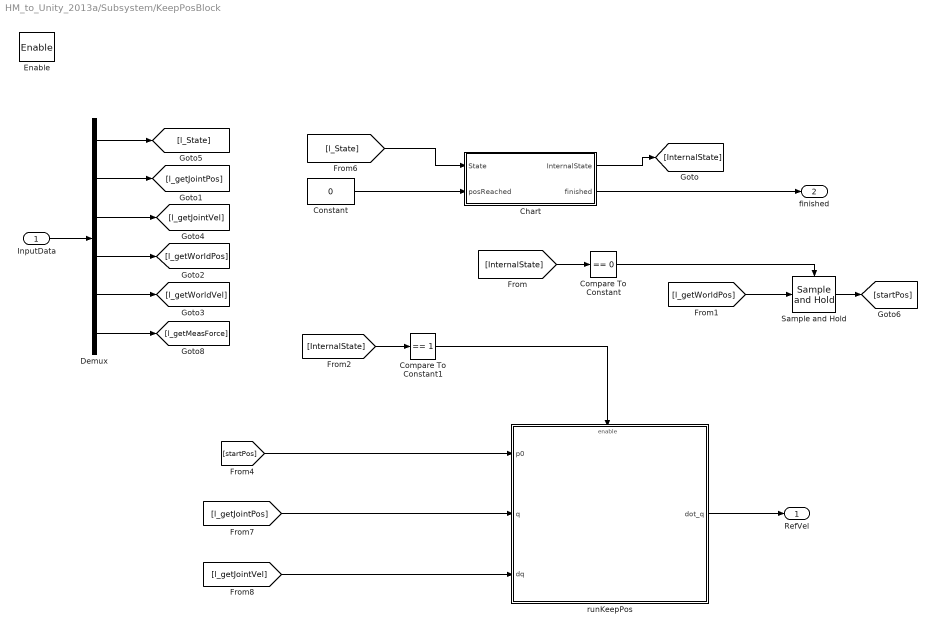
== system HM_to_Unity_2013a/Subsystem/KeepPosBlock ==
  InputData : Inport
  Enable : EnablePort  StatesWhenEnabling=reset
  Chart : Stateflow chart  TreatAsAtomicUnit=on
  Compare To Constant : simulink/Logic and Bit Operations/Compare To Constant  relop===  const=0  OutDataTypeStr=uint8  ZeroCross=off
  Compare To Constant1 : simulink/Logic and Bit Operations/Compare To Constant  relop===  const=1  OutDataTypeStr=uint8  ZeroCross=off
  Constant : Constant  Value=0
  Demux : Demux  Outputs=[1 3 3 3 3 3]
  Sample and Hold : dspsigops/Sample and Hold  trig=Rising edge  initCond=[0 0 0]  latchinput=off
  runKeepPos : Subsystem  TreatAsAtomicUnit=on
  RefVel : Outport  InitialOutput=[0 0 0]
  finished : Outport  Port=2  OutDataTypeStr=boolean  OutputWhenDisabled=reset  InitialOutput=0
  wires:
  Sample and Hold/1 -> [startPos]
  [InternalState] -> Compare To Constant/1
  Compare To Constant/1 -> Sample and Hold/Trigger
  [InternalState] -> Compare To Constant1/1
  Compare To Constant1/1 -> runKeepPos/Enable
  [startPos] -> runKeepPos/1(p0)
  Chart/1(InternalState) -> [InternalState]
  [l_getWorldPos] -> Sample and Hold/1
  [l_State] -> Chart/1(State)
  runKeepPos/1(dot_q) -> RefVel/1
  [l_getJointPos] -> runKeepPos/2(q)
  [l_getJointVel] -> runKeepPos/3(dq)
  Chart/2(finished) -> finished/1
  Constant/1 -> Chart/2(posReached)
  InputData/1 -> Demux/1
  Demux/1 -> [l_State]
  Demux/2 -> [l_getJointPos]
  Demux/3 -> [l_getJointVel]
  Demux/4 -> [l_getWorldPos]
  Demux/5 -> [l_getWorldVel]
  Demux/6 -> [l_getMeasForce]

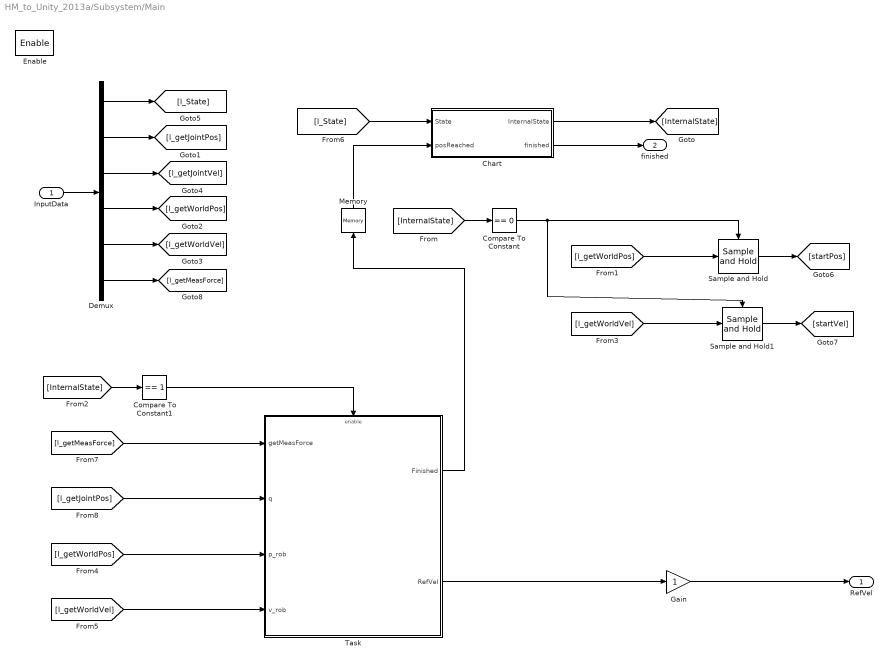
== system HM_to_Unity_2013a/Subsystem/Main ==
  InputData : Inport
  Enable : EnablePort  StatesWhenEnabling=reset
  Chart : Stateflow chart  TreatAsAtomicUnit=on
  Compare To Constant : simulink/Logic and Bit Operations/Compare To Constant  relop===  const=0  OutDataTypeStr=uint8  ZeroCross=off
  Compare To Constant1 : simulink/Logic and Bit Operations/Compare To Constant  relop===  const=1  OutDataTypeStr=uint8  ZeroCross=off
  Demux : Demux  Outputs=[1 3 3 3 3 3]
  Gain : Gain
  Memory : Memory  InheritSampleTime=on
  Sample and Hold : dspsigops/Sample and Hold  trig=Rising edge  initCond=[0 0 0]  latchinput=off
  Sample and Hold1 : dspsigops/Sample and Hold  trig=Rising edge  initCond=[0 0 0]  latchinput=off
  Task : Subsystem
  RefVel : Outport  InitialOutput=[0 0 0]
  finished : Outport  Port=2  OutDataTypeStr=boolean  OutputWhenDisabled=reset  InitialOutput=0
  wires:
  InputData/1 -> Demux/1
  Demux/1 -> [l_State]
  Demux/2 -> [l_getJointPos]
  Demux/3 -> [l_getJointVel]
  Demux/4 -> [l_getWorldPos]
  Demux/5 -> [l_getWorldVel]
  Sample and Hold/1 -> [startPos]
  [InternalState] -> Compare To Constant/1
  Compare To Constant/1 -> Sample and Hold/Trigger, Sample and Hold1/Trigger
  [InternalState] -> Compare To Constant1/1
  [l_getWorldVel] -> Sample and Hold1/1
  Sample and Hold1/1 -> [startVel]
  Chart/1(InternalState) -> [InternalState]
  [l_getWorldPos] -> Sample and Hold/1
  [l_State] -> Chart/1(State)
  Chart/2(finished) -> finished/1
  Compare To Constant1/1 -> Task/Enable
  Memory/1 -> Chart/2(posReached)
  [l_getJointPos] -> Task/2(q)
  Gain/1 -> RefVel/1
  Task/2(RefVel) -> Gain/1
  [l_getWorldPos] -> Task/3(p_rob)
  [l_getWorldVel] -> Task/4(v_rob)
  Task/1(Finished) -> Memory/1
  Demux/6 -> [l_getMeasForce]
  [l_getMeasForce] -> Task/1(getMeasForce)

== system HM_to_Unity_2013a/HapticMaster inputs/Balanca enkoderji/Desna roka ==
  Rst : Inport
  JR3 Input : sensors_jr3_lib/Auxiliary blocks/JR3 Input  board=0  dsp=1  filter=0  fullscale=[150 150 300 8 8 8]  sampletime=0.0004
  SH : dspsigops/Sample and Hold  trig=Rising edge  initCond=[0 0 0 0 0 0]  latchinput=off
  Selector : Selector  InputPortWidth=6  IndexOptions=Index vector (dialog)  Indices="[1  2  3]"  OutputSizes=1
  Sum : Sum  Inputs=-+|
  FT : Outport
  wires:
  Selector/1 -> FT/1
  Sum/1 -> Selector/1
  SH/1 -> Sum/1
  JR3 Input/1 -> Sum/2, SH/1
  Rst/1 -> SH/Trigger

== system HM_to_Unity_2013a/Robot State Control/Subsystem8/Subsystem ==
  In1 : Inport
  Compare To Constant : simulink/Logic and Bit Operations/Compare To Constant  relop=>  const=0.004  OutDataTypeStr=uint8  ZeroCross=off
  Data Type Conversion : DataTypeConversion  OutDataTypeStr=double
  Discrete-Time Integrator : DiscreteIntegrator  ExternalReset=either  SampleTime=-1  LimitOutput=on  UpperSaturationLimit=1  LowerSaturationLimit=0  ICPrevOutput=DiscIntNeverNeededParam  ICPrevScaledInput=DiscIntNeverNeededParam
  Out1 : Outport
  wires:
  Discrete-Time Integrator/1 -> Compare To Constant/1
  In1/1 -> Discrete-Time Integrator/1, Discrete-Time Integrator/2
  Compare To Constant/1 -> Data Type Conversion/1
  Data Type Conversion/1 -> Out1/1

== system HM_to_Unity_2013a/Robot State Control/Subsystem8/Subsystem1 ==
  In1 : Inport
  Compare To Constant : simulink/Logic and Bit Operations/Compare To Constant  relop=>  const=0.004  OutDataTypeStr=uint8  ZeroCross=off
  Data Type Conversion : DataTypeConversion  OutDataTypeStr=double
  Discrete-Time Integrator : DiscreteIntegrator  ExternalReset=either  SampleTime=-1  LimitOutput=on  UpperSaturationLimit=1  LowerSaturationLimit=0  ICPrevOutput=DiscIntNeverNeededParam  ICPrevScaledInput=DiscIntNeverNeededParam
  Out1 : Outport
  wires:
  Compare To Constant/1 -> Data Type Conversion/1
  In1/1 -> Discrete-Time Integrator/2, Discrete-Time Integrator/1
  Discrete-Time Integrator/1 -> Compare To Constant/1
  Data Type Conversion/1 -> Out1/1

== system HM_to_Unity_2013a/Robot State Control/Subsystem8/Subsystem2 ==
  In1 : Inport
  Compare To Constant : simulink/Logic and Bit Operations/Compare To Constant  relop=>  const=0.004  OutDataTypeStr=uint8  ZeroCross=off
  Data Type Conversion : DataTypeConversion  OutDataTypeStr=double
  Discrete-Time Integrator : DiscreteIntegrator  ExternalReset=either  SampleTime=-1  LimitOutput=on  UpperSaturationLimit=1  LowerSaturationLimit=0  ICPrevOutput=DiscIntNeverNeededParam  ICPrevScaledInput=DiscIntNeverNeededParam
  Out1 : Outport
  wires:
  Discrete-Time Integrator/1 -> Compare To Constant/1
  In1/1 -> Discrete-Time Integrator/1, Discrete-Time Integrator/2
  Compare To Constant/1 -> Data Type Conversion/1
  Data Type Conversion/1 -> Out1/1

== system HM_to_Unity_2013a/Robot State Control/Subsystem8/Subsystem3 ==
  In1 : Inport
  Compare To Constant : simulink/Logic and Bit Operations/Compare To Constant  relop=>  const=0.004  OutDataTypeStr=uint8  ZeroCross=off
  Data Type Conversion : DataTypeConversion  OutDataTypeStr=double
  Discrete-Time Integrator : DiscreteIntegrator  ExternalReset=either  SampleTime=-1  LimitOutput=on  UpperSaturationLimit=1  LowerSaturationLimit=0  ICPrevOutput=DiscIntNeverNeededParam  ICPrevScaledInput=DiscIntNeverNeededParam
  Out1 : Outport
  wires:
  Compare To Constant/1 -> Data Type Conversion/1
  In1/1 -> Discrete-Time Integrator/2, Discrete-Time Integrator/1
  Discrete-Time Integrator/1 -> Compare To Constant/1
  Data Type Conversion/1 -> Out1/1

== system HM_to_Unity_2013a/Robot State Control/Subsystem8/Subsystem4 ==
  In1 : Inport
  Compare To Constant : simulink/Logic and Bit Operations/Compare To Constant  relop=>  const=0.004  OutDataTypeStr=uint8  ZeroCross=off
  Data Type Conversion : DataTypeConversion  OutDataTypeStr=double
  Discrete-Time Integrator : DiscreteIntegrator  ExternalReset=either  SampleTime=-1  LimitOutput=on  UpperSaturationLimit=1  LowerSaturationLimit=0  ICPrevOutput=DiscIntNeverNeededParam  ICPrevScaledInput=DiscIntNeverNeededParam
  Out1 : Outport
  wires:
  Data Type Conversion/1 -> Out1/1
  Compare To Constant/1 -> Data Type Conversion/1
  In1/1 -> Discrete-Time Integrator/2, Discrete-Time Integrator/1
  Discrete-Time Integrator/1 -> Compare To Constant/1

== system HM_to_Unity_2013a/Robot State Control/Subsystem8/Subsystem5 ==
  In1 : Inport
  Compare To Constant : simulink/Logic and Bit Operations/Compare To Constant  relop=>  const=0.004  OutDataTypeStr=uint8  ZeroCross=off
  Data Type Conversion : DataTypeConversion  OutDataTypeStr=double
  Discrete-Time Integrator : DiscreteIntegrator  ExternalReset=either  SampleTime=-1  LimitOutput=on  UpperSaturationLimit=1  LowerSaturationLimit=0  ICPrevOutput=DiscIntNeverNeededParam  ICPrevScaledInput=DiscIntNeverNeededParam
  Out1 : Outport
  wires:
  Discrete-Time Integrator/1 -> Compare To Constant/1
  In1/1 -> Discrete-Time Integrator/1, Discrete-Time Integrator/2
  Compare To Constant/1 -> Data Type Conversion/1
  Data Type Conversion/1 -> Out1/1

== system HM_to_Unity_2013a/Robot State Control/Subsystem8/Subsystem6 ==
  In1 : Inport
  Compare To Constant : simulink/Logic and Bit Operations/Compare To Constant  relop=>  const=0.004  OutDataTypeStr=uint8  ZeroCross=off
  Data Type Conversion : DataTypeConversion  OutDataTypeStr=double
  Discrete-Time Integrator : DiscreteIntegrator  ExternalReset=either  SampleTime=-1  LimitOutput=on  UpperSaturationLimit=1  LowerSaturationLimit=0  ICPrevOutput=DiscIntNeverNeededParam  ICPrevScaledInput=DiscIntNeverNeededParam
  Out1 : Outport
  wires:
  Data Type Conversion/1 -> Out1/1
  Compare To Constant/1 -> Data Type Conversion/1
  In1/1 -> Discrete-Time Integrator/2, Discrete-Time Integrator/1
  Discrete-Time Integrator/1 -> Compare To Constant/1

== system HM_to_Unity_2013a/Robot State Control/Subsystem8/Subsystem7 ==
  In1 : Inport
  Compare To Constant : simulink/Logic and Bit Operations/Compare To Constant  relop=>  const=0.004  OutDataTypeStr=uint8  ZeroCross=off
  Data Type Conversion : DataTypeConversion  OutDataTypeStr=double
  Discrete-Time Integrator : DiscreteIntegrator  ExternalReset=either  SampleTime=-1  LimitOutput=on  UpperSaturationLimit=1  LowerSaturationLimit=0  ICPrevOutput=DiscIntNeverNeededParam  ICPrevScaledInput=DiscIntNeverNeededParam
  Out1 : Outport
  wires:
  Discrete-Time Integrator/1 -> Compare To Constant/1
  In1/1 -> Discrete-Time Integrator/1, Discrete-Time Integrator/2
  Compare To Constant/1 -> Data Type Conversion/1
  Data Type Conversion/1 -> Out1/1

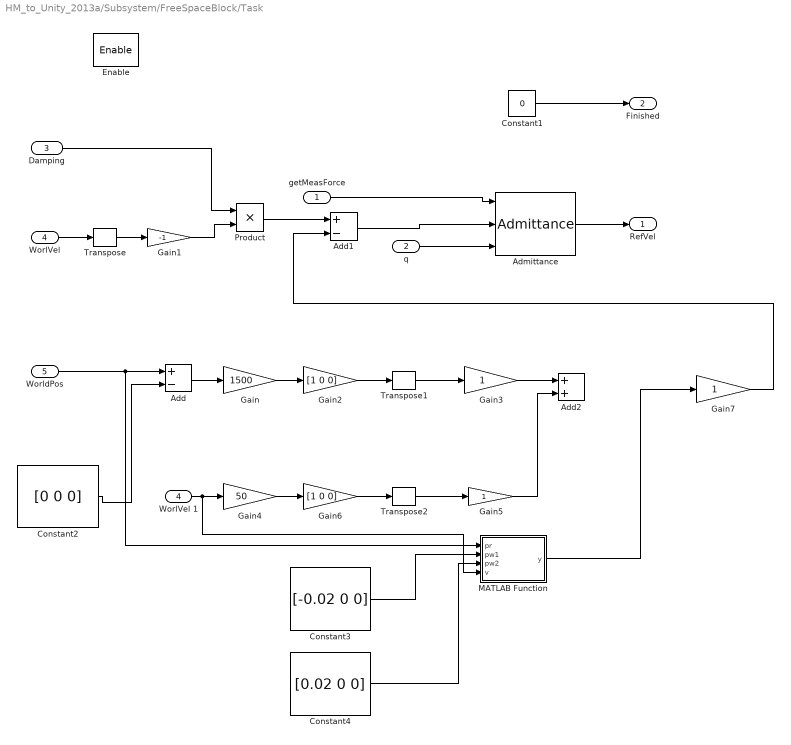
== system HM_to_Unity_2013a/Subsystem/FreeSpaceBlock/Task ==
  getMeasForce : Inport
  q : Inport  Port=2
  Damping : Inport  Port=3  OutMin=0  OutMax=250
  "WorlVel " : Inport  Port=4
  WorldPos : Inport  Port=5
  Enable : EnablePort  StatesWhenEnabling=reset
  Add : Sum  Inputs=+-
  Add1 : Sum  Inputs=+-
  Add2 : Sum
  "Admittance " : hm_control_lib/Admittance   MassRobotTop=3  Acceleration_limit=[100 100 100]  Velocity_limit=[0.7 0.3 0.3]
  Constant1 : Constant  Value=0
  Constant2 : Constant  Value=[0 0 0]  SampleTime=-1
  Constant3 : Constant  Value=[-0.02 0 0]  SampleTime=-1
  Constant4 : Constant  Value=[0.02 0 0]  SampleTime=-1
  Gain : Gain  Gain=1500
  Gain1 : Gain  Gain=-1
  Gain2 : Gain  Gain=[1 0 0]
  Gain3 : Gain
  Gain4 : Gain  Gain=50
  Gain5 : Gain
  Gain6 : Gain  Gain=[1 0 0]
  Gain7 : Gain
  MATLAB Function : MATLAB Function  TreatAsAtomicUnit=on
  Product : Product
  Transpose : dspmtrx3/Transpose  Hermitian=off  overflowFlag=off
  Transpose1 : dspmtrx3/Transpose  Hermitian=off  overflowFlag=off
  Transpose2 : dspmtrx3/Transpose  Hermitian=off  overflowFlag=off
  WorlVel 1 : InportShadow  Port=4
  RefVel : Outport  InitialOutput=[0 0 0]
  Finished : Outport  Port=2  InitialOutput=[0]
  wires:
  "Admittance "/1 -> RefVel/1
  getMeasForce/1 -> "Admittance "/1
  q/1 -> "Admittance "/3
  Constant1/1 -> Finished/1
  Gain1/1 -> Product/2
  Damping/1 -> Product/1
  "WorlVel "/1 -> Transpose/1
  Transpose/1 -> Gain1/1
  WorldPos/1 -> MATLAB Function/1(pr), Add/1
  Constant2/1 -> Add/2
  Add/1 -> Gain/1
  Gain/1 -> Gain2/1
  Product/1 -> Add1/1
  Add1/1 -> "Admittance "/2
  Gain2/1 -> Transpose1/1
  Transpose1/1 -> Gain3/1
  Transpose2/1 -> Gain5/1
  Gain4/1 -> Gain6/1
  Gain3/1 -> Add2/1
  Gain5/1 -> Add2/2
  WorlVel 1/1 -> MATLAB Function/4(v), Gain4/1
  Gain6/1 -> Transpose2/1
  Gain7/1 -> Add1/2
  Constant4/1 -> MATLAB Function/3(pw2)
  Constant3/1 -> MATLAB Function/2(pw1)
  MATLAB Function/1(y) -> Gain7/1

== system HM_to_Unity_2013a/Subsystem/GotoBlock/runGoTo ==
  p0 : Inport
  v0 : Inport  Port=2
  pk : Inport  Port=3
  vk : Inport  Port=4
  T : Inport  Port=5
  q : Inport  Port=6
  dq : Inport  Port=7
  Sample time : Inport  Port=8
  Enable : EnablePort  StatesWhenEnabling=reset
  Counter Free-Running : simulink/Sources/Counter Free-Running  NumBits=16  tsamp=-1
  Data Type Conversion : DataTypeConversion  OutDataTypeStr=double
  Embedded MATLAB Function : MATLAB Function  TreatAsAtomicUnit=on
  HapticMaster InverseKinematics : S-Function  InitFcn=try, set_param(gcb,'FunctionName','HM_InverseKinematics'), end  FunctionName=HM_InverseKinematics  SFunctionModules=HM_InverseKinematics_wrapper  EnableBusSupport=off  mask(S-Function Builder){}
      mask help: The S-Function Builder block creates a wrapper C-MEX S-function from your supplied C code with multiple input ports, output ports, and a variable number of scalar, vector, or matrix parameters. The input and output ports can propagate Simulink built-in data types, fixed-point datatypes, complex, frame, 1-D, and 2-D signals. This block also supports discrete and continuous states of type real. You can optionally have the block generate a TLC file to be used with Real-Time Workshop for code generation.
      mask init: same as HM_to_Unity_2013a/HapticMaster inputs/HapticMaster DirectKinematics T1
      settings: CopyFcn=set_param(gcbh,'LinkStatus','none')  PreSaveFcn=try, set_param(gcb,'FunctionName','HM_InverseKinematics'), end  OpenFcn=sfunctionwizard(gcbh)
      mask Display:
      | plot(val(:,1),val(:,2)),disp(sys)
      | port_label('input',1,'x')
      | port_label('output',1,'q')
  Product : Product  RndMeth=Zero
  Subsystem : Subsystem  mask{Differetial_gain=[0.1 0.1 0.1], Proportional_gain=[100 100 100]}
  Terminator : Terminator
  dot_q : Outport  OutputWhenDisabled=reset  InitialOutput=[0 0 0]
  wires:
  p0/1 -> Embedded MATLAB Function/1(p0)
  Counter Free-Running/1 -> Data Type Conversion/1
  Data Type Conversion/1 -> Product/1
  Sample time/1 -> Product/2
  Product/1 -> Embedded MATLAB Function/6(t)
  v0/1 -> Embedded MATLAB Function/2(v0)
  pk/1 -> Embedded MATLAB Function/3(pk)
  vk/1 -> Embedded MATLAB Function/4(vk)
  T/1 -> Embedded MATLAB Function/5(T)
  Subsystem/1(dot_q) -> dot_q/1
  Embedded MATLAB Function/1(p) -> HapticMaster InverseKinematics/1
  q/1 -> Subsystem/2(q_ac)
  dq/1 -> Subsystem/3(dot_q_ac)
  Embedded MATLAB Function/2(v) -> Terminator/1
  HapticMaster InverseKinematics/1 -> Subsystem/1(q_des)

== system HM_to_Unity_2013a/Subsystem/KeepPosBlock/runKeepPos ==
  p0 : Inport
  q : Inport  Port=2
  dq : Inport  Port=3
  Enable : EnablePort  StatesWhenEnabling=reset
  HapticMaster InverseKinematics : S-Function  InitFcn=try, set_param(gcb,'FunctionName','HM_InverseKinematics'), end  FunctionName=HM_InverseKinematics  SFunctionModules=HM_InverseKinematics_wrapper  EnableBusSupport=off  mask(S-Function Builder){}
      mask help: The S-Function Builder block creates a wrapper C-MEX S-function from your supplied C code with multiple input ports, output ports, and a variable number of scalar, vector, or matrix parameters. The input and output ports can propagate Simulink built-in data types, fixed-point datatypes, complex, frame, 1-D, and 2-D signals. This block also supports discrete and continuous states of type real. You can optionally have the block generate a TLC file to be used with Real-Time Workshop for code generation.
      mask init: same as HM_to_Unity_2013a/HapticMaster inputs/HapticMaster DirectKinematics T1
      settings: CopyFcn=set_param(gcbh,'LinkStatus','none')  PreSaveFcn=try, set_param(gcb,'FunctionName','HM_InverseKinematics'), end  OpenFcn=sfunctionwizard(gcbh)
      mask Display:
      | plot(val(:,1),val(:,2)),disp(sys)
      | port_label('input',1,'x')
      | port_label('output',1,'q')
  Subsystem : Subsystem  mask{Differetial_gain=[0.1 0.1 0.1], Proportional_gain=[100 100 100]}
  dot_q : Outport
  wires:
  Subsystem/1(dot_q) -> dot_q/1
  p0/1 -> HapticMaster InverseKinematics/1
  q/1 -> Subsystem/2(q_ac)
  dq/1 -> Subsystem/3(dot_q_ac)
  HapticMaster InverseKinematics/1 -> Subsystem/1(q_des)

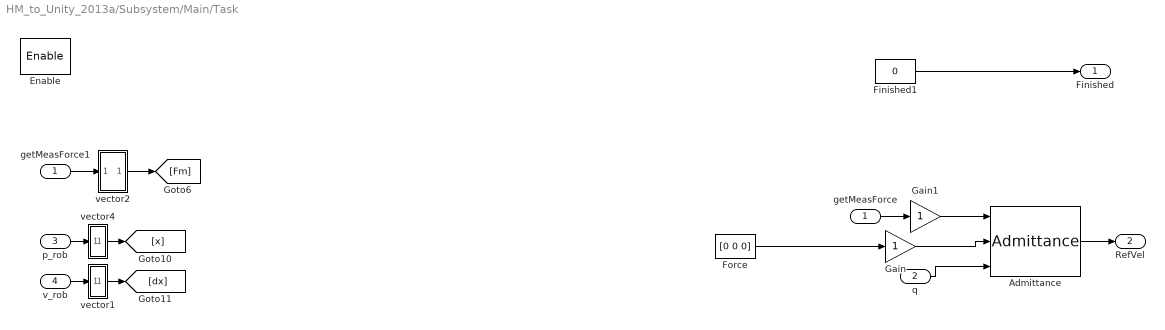
== system HM_to_Unity_2013a/Subsystem/Main/Task ==
  getMeasForce : Inport
  q : Inport  Port=2
  p_rob : Inport  Port=3
  v_rob : Inport  Port=4
  Enable : EnablePort
  "Admittance " : hm_control_lib/Admittance   MassRobotTop=2  Acceleration_limit=[100 100 100]  Velocity_limit=[0.7 0.3 0.3]
  Finished1 : Constant  Value=0
  Force : Constant  Value=[0 0 0]
  Gain : Gain
  Gain1 : Gain
  getMeasForce1 : InportShadow
  vector1 : MATLAB Function  TreatAsAtomicUnit=on
  vector2 : MATLAB Function  TreatAsAtomicUnit=on
  vector4 : MATLAB Function  TreatAsAtomicUnit=on
  Finished : Outport
  RefVel : Outport  Port=2
  wires:
  getMeasForce/1 -> Gain1/1
  q/1 -> "Admittance "/3
  Gain/1 -> "Admittance "/2
  Gain1/1 -> "Admittance "/1
  p_rob/1 -> vector4/1(u)
  v_rob/1 -> vector1/1(u)
  Finished1/1 -> Finished/1
  "Admittance "/1 -> RefVel/1
  vector4/1(y) -> [x]
  vector1/1(y) -> [dx]
  getMeasForce1/1 -> vector2/1(u)
  vector2/1(y) -> [Fm]
  Force/1 -> Gain/1

== system HM_to_Unity_2013a/Subsystem/GotoBlock/runGoTo/Subsystem ==
  q_des : Inport
  q_ac : Inport  Port=2
  dot_q_ac : Inport  Port=3
  Add : Sum  Inputs=-+|
  Add1 : Sum  Inputs=-+|
  Kd : Gain  Gain=[Differetial_gain(1) Differetial_gain(2) Differetial_gain(3)]
  Kp : Gain  Gain=[Proportional_gain(1) Proportional_gain(2) Proportional_gain(3)]
  dot_q : Outport
  wires:
  q_ac/1 -> Add/1
  Kd/1 -> Add1/1
  Add1/1 -> dot_q/1  "dot_q"
  Kp/1 -> Add1/2
  Add/1 -> Kp/1
  q_des/1 -> Add/2
  dot_q_ac/1 -> Kd/1

== system HM_to_Unity_2013a/Subsystem/KeepPosBlock/runKeepPos/Subsystem ==
  q_des : Inport
  q_ac : Inport  Port=2
  dot_q_ac : Inport  Port=3
  Add : Sum  Inputs=-+|
  Add1 : Sum  Inputs=-+|
  Kd : Gain  Gain=[Differetial_gain(1) Differetial_gain(2) Differetial_gain(3)]
  Kp : Gain  Gain=[Proportional_gain(1) Proportional_gain(2) Proportional_gain(3)]
  dot_q : Outport
  wires:
  q_ac/1 -> Add/1
  Kd/1 -> Add1/1
  Add1/1 -> dot_q/1  "dot_q"
  Kp/1 -> Add1/2
  Add/1 -> Kp/1
  q_des/1 -> Add/2
  dot_q_ac/1 -> Kd/1

== matlab function HM_to_Unity_2013a/Subsystem/FreeSpaceBlock/Task/MATLAB Function ==
  data: pr input; y output; pw1 input; pw2 input; v input
function y = fcn(pr, pw1, pw2, v)
%#codegen
k = 1500;
b = 50;
Fw1 = 0;
Fw2 = 0;
Fd = b*v(1);

if(pr(1)<pw1(1))
Fw1 = -k*(pw1(1)-pr(1))+Fd;
end 

if(pr(1)>pw2(1))
Fw2 = -k*(pw2(1)-pr(1))+Fd;
end
y = [Fw1+Fw2,0,0]';

== stateflow chart HM_to_Unity_2013a/Subsystem/FreeSpaceBlock/Chart ==
  state Inactive
    en:InternalState=-1;
  state Init
    en:InternalState=0;
    finished=0;
  state Running
    du:InternalState=1;
  state positionReached
    en:InternalState=2;
    finished=1;
  (default) -> Inactive
  Inactive -> Init : [State==1]
  Init -> Running : [InternalState==0]
  Running -> positionReached : [posReached==1]
  data: State input; InternalState output double; posReached input; finished output boolean

== stateflow chart HM_to_Unity_2013a/Subsystem/Main/Chart ==
  state Inactive
    en:InternalState=-1;
  state Init
    en:InternalState=0;
    finished=0;
  state Running
    du:InternalState=1;
  state positionReached
    en:InternalState=2;
    finished=1;
  (default) -> Inactive
  Inactive -> Init : [State==2]
  Init -> Running : [InternalState==0]
  Running -> positionReached : [posReached==1]
  data: State input; InternalState output double; posReached input; finished output boolean

== stateflow chart HM_to_Unity_2013a/Subsystem/GotoBlock/Chart ==
  state Inactive
    en:InternalState=-1;
  state Init
    en:InternalState=0;
    finished=0;
  state Running
    du:InternalState=1;
  state positionReached
    en:InternalState=2;
    finished=1;
  (default) -> Inactive
  Inactive -> Init : [State==3]
  Init -> Running : [InternalState==0]
  Running -> positionReached : [posReached==1]
  data: State input; InternalState output double; posReached input; finished output boolean
